simulink model "sim_udp_realtime"  (R2022b)
settings: Solver=FixedStepAuto  StartTime=0.0  StopTime=10.0  FixedStep=param_global.Ta  RelTol=1e-3
libraries: dspnetwork x2
settings Model: Creator=emu  LastModifiedBy=emu

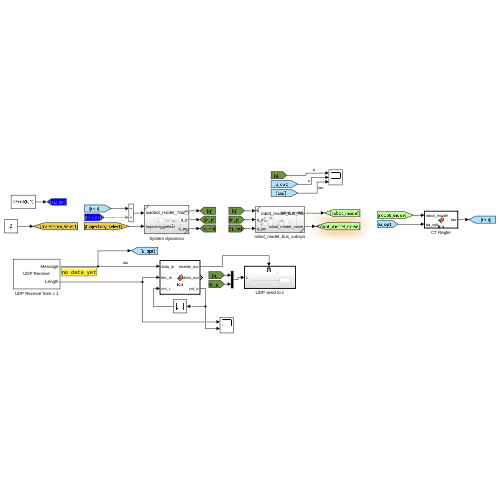
[thumbnail: Simulink's stored preview of the top-level diagram]
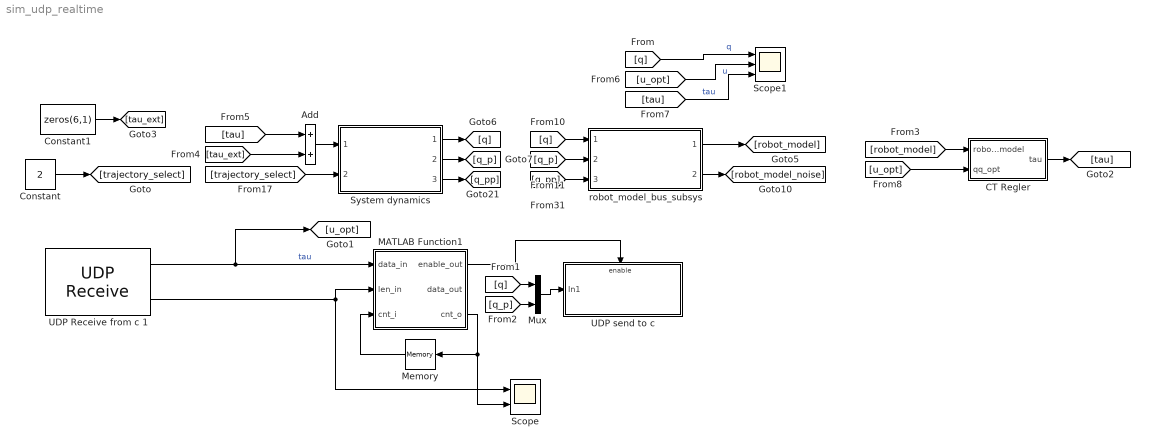
== system sim_udp_realtime ==
  Add : Sum
  CT Regler : MATLAB Function  TreatAsAtomicUnit=on
  Constant : Constant  Value=2
  Constant1 : Constant  Value=zeros(6,1)
  MATLAB Function1 : MATLAB Function  TreatAsAtomicUnit=on
  Memory : Memory
  Mux : Mux  Inputs=2
  Scope : Scope  NumInputPorts=2
  Scope1 : Scope  NumInputPorts=3
  System dynamics : Subsystem  ReferencedSubsystem=robot_model_7dof_ref_subsys
  UDP Receive from c 1 : dspnetwork/UDP Receive  localURL='0.0.0.0'  localPort=8080  remoteURL='127.0.0.1'  remotePort=-1  recvBufferSize=48  dims=6  signalDatatype=double  isComplex=off  isVarSize=off  showBlockingTime=off  blockingTime=0  sampletime=param_global.Ta  blockPlatform=[]
      settings: LibrarySourceBlock=dspsrcs4/UDP Receive
  UDP send to c : Subsystem
  robot_model_bus_subsys : Subsystem  ReferencedSubsystem=robot_model_bus_7dof_ref_subsys
  wires:
  UDP Receive from c 1/1 -> [u_opt], MATLAB Function1/1(data_in)  "tau"
  UDP Receive from c 1/2 -> Scope/1, MATLAB Function1/2(len_in)
  MATLAB Function1/1(enable_out) -> UDP send to c/Enable
  MATLAB Function1/3(cnt_o) -> Scope/2, Memory/1
  Memory/1 -> MATLAB Function1/3(cnt_i)
  System dynamics/2 -> [q_p]
  [tau_ext] -> Add/2
  System dynamics/3 -> [q_pp]
  System dynamics/1 -> [q]
  [tau] -> Add/1
  Add/1 -> System dynamics/1
  [trajectory_select] -> System dynamics/2
  Constant/1 -> [trajectory_select]
  [q] -> Scope1/1  "q"
  [q_p] -> robot_model_bus_subsys/2
  [q_pp] -> robot_model_bus_subsys/3
  robot_model_bus_subsys/1 -> [robot_model]
  [q] -> robot_model_bus_subsys/1
  robot_model_bus_subsys/2 -> [robot_model_noise]
  [u_opt] -> CT Regler/2(qq_opt)
  [robot_model] -> CT Regler/1(robot_model)
  CT Regler/1(tau) -> [tau]
  [q] -> Mux/1
  [q_p] -> Mux/2
  Mux/1 -> UDP send to c/1(In1)
  Constant1/1 -> [tau_ext]
  [u_opt] -> Scope1/2  "u"
  [tau] -> Scope1/3  "tau"

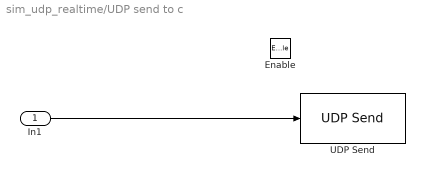
== system sim_udp_realtime/UDP send to c ==
  In1 : Inport
  Enable : EnablePort
  UDP Send : dspnetwork/UDP Send  remoteURL='127.0.0.1'  remotePort=8081  localURL='0.0.0.0'  localPortSource=Automatically determine  localPort=8081  sendBufferSize=96  sampletime=-1  blockPlatform=[]  separateLengthPort=0
      settings: LibrarySourceBlock=dspsnks4/UDP Send
  wires:
  In1/1 -> UDP Send/1

== matlab function sim_udp_realtime/MATLAB Function1 ==
  settings: updateMethod=DISCRETE  sampleTime=param_global.Ta
  data: enable_out output; data_in input; len_in input; data_out output; cnt_i input; cnt_o output
function [enable_out, data_out, cnt_o] = fcn(data_in, len_in, cnt_i)

if(len_in > 0)
    cnt_o = cnt_i + 1;
else
    cnt_o = cnt_i;
end

enable_out = 1;
data_out = [-0.0349; -2.4613; -3.5569; 2.2398; 0.0350; -1.2488; 1; 2; 3; 4; 5; 6];

== matlab function sim_udp_realtime/CT Regler ==
  data: robot_model input Bus: robot_model; tau output; qq_opt input
function tau = fcn(robot_model, qq_opt)

if size(qq_opt, 2) ~= 0 && size(qq_opt, 1) ~= 1
    q_d_pp = qq_opt;

    M = robot_model.M;      % inertia matrix
    C_rnea = robot_model.C_rnea; % C_rnea(q, q_p) = C(q, q_p)q_p + g(q) = n(q, q_p)
    
    tau = M*q_d_pp + C_rnea;
else
    tau = zeros(6,1);
end
